simulink model "FlightSimulation"  (R2025b)
settings: Solver=ode3  StartTime=0.0  StopTime=100  FixedStep=params.time.dt  RelTol=1e-3
values from neighbouring files (symbols this model uses):
  launch_ECEF_m = lla2ecef(launchLLA)    [RunSim.m]    (also in RunSimulink.m)
  launchAlt = 180    [RunSim.m]    (also in RunSimulink.m = 10)
  launchLLA = [launchLat, launchLon, launchAlt]    [RunSim.m]    (also in RunSimulink.m)
  q = q / norm(q)    [CorrectQuaternionKinematics.m]    (also in solveLQR.m = 0.5*rho*vel^2)
  q_TB_0 = dcm2quat(R_TB_0)    [RunSimulink.m]
  w_ib_x = 0.00    (= 0)    [RunSim.m]    (also in RunSimulink.m = 1e-10)
  w_ib_y = 0.00    (= 0)    [RunSim.m]    (also in RunSimulink.m = 1e-10)
  w_ib_z = 0.00    (= 0)    [RunSim.m]    (also in RunSimulink.m = 1e-10)
undefined symbols (not defined in the file or in its folder): Earth, F, kfConsts, kfErrInds, kfInds, launchGeoidHeight, Light, MIL, nav_covs, nav_state, params, WGS84, WMM2025
libraries: simulink x6, aerolibatmos2 x5, aerolibgravity2 x3, aerolib6dof2 x1, aerolibwind2 x1, simulink_extras x1, matrix_library x1, aerolibtransform2 x1, lib_utils x1
(part 1 of 2)
settings Model: Creator=pearsdj1  LastModifiedBy=abhay

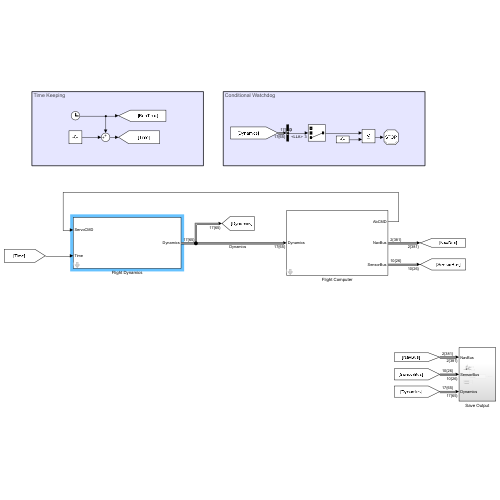
[thumbnail: Simulink's stored preview of the top-level diagram]
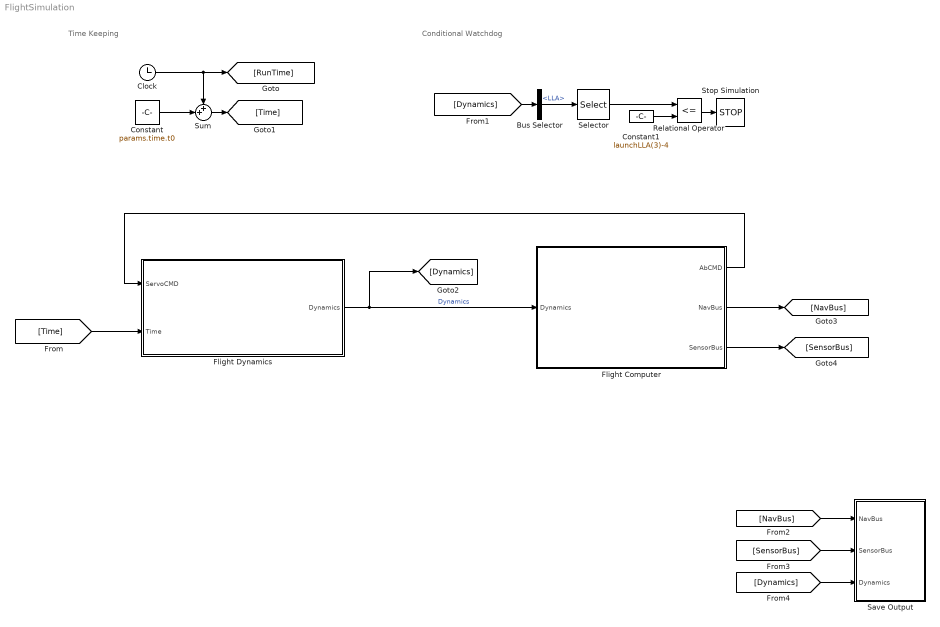
== system FlightSimulation ==
  note: Time Keeping
  note: Conditional Watchdog
  Bus Selector : BusSelector  OutputSignals=LLA
  Clock : Clock
  Constant : Constant  Value=params.time.t0
  Constant1 : Constant  Value=launchLLA(3)-4
  Flight Computer : Subsystem  mask{navParams=params.navParams, navInds=params.navInds, navConst=params.navConst, const=params.const, time=params.time}
      mask prompts: navParams "Navigator Params"; navInds "Navigator Indices"; navConst "Navigator Constants"; const "Constants"
      mask DialogControl DescGroupVar Prompt: Flight Computer
      mask DialogControl DescTextVar Prompt: Here lies the flight computer, with stuff and things ya'know
      mask DialogControl ParameterGroupVar Prompt: Navigator Parameters
  Flight Dynamics : Subsystem  mask{MotorModel=params.MotorModel, kins=params.kins, AeroModel=params.AeroModel, const=params.const}
      mask prompts: MotorModel "Motor Model"; kins "Kinematic Model"; AeroModel "Aerodynamic Model"; const "Constants"
      mask DialogControl DescGroupVar Prompt: Flight Dynamics
      mask DialogControl DescTextVar Prompt: Here be the dynamics of Sir Archimedes, according to all known laws of aviation...
  Relational Operator : RelationalOperator  Operator=<=  OutDataTypeStr=boolean  RndMeth=Simplest  InputSameDT=off
  Save Output : Subsystem
  Selector : Selector  InputPortWidth=3  IndexOptions=Index vector (dialog)  Indices=3  OutputSizes=1
  Stop Simulation : Stop
  Sum : Sum  Inputs=++|
  wires:
  Constant/1 -> Sum/2
  Clock/1 -> Sum/1, [RunTime]
  Sum/1 -> [Time]
  Flight Dynamics/1(Dynamics) -> [Dynamics], Flight Computer/1(Dynamics)  "Dynamics"
  Flight Computer/2(NavBus) -> [NavBus]
  Flight Computer/3(SensorBus) -> [SensorBus]
  [Time] -> Flight Dynamics/2(Time)
  Flight Computer/1(AbCMD) -> Flight Dynamics/1(ServoCMD)
  Constant1/1 -> Relational Operator/2
  [Dynamics] -> Bus Selector/1
  Bus Selector/1 -> Selector/1  "<LLA>"
  Selector/1 -> Relational Operator/1
  Relational Operator/1 -> Stop Simulation/1
  [NavBus] -> Save Output/1(NavBus)
  [SensorBus] -> Save Output/2(SensorBus)
  [Dynamics] -> Save Output/3(Dynamics)

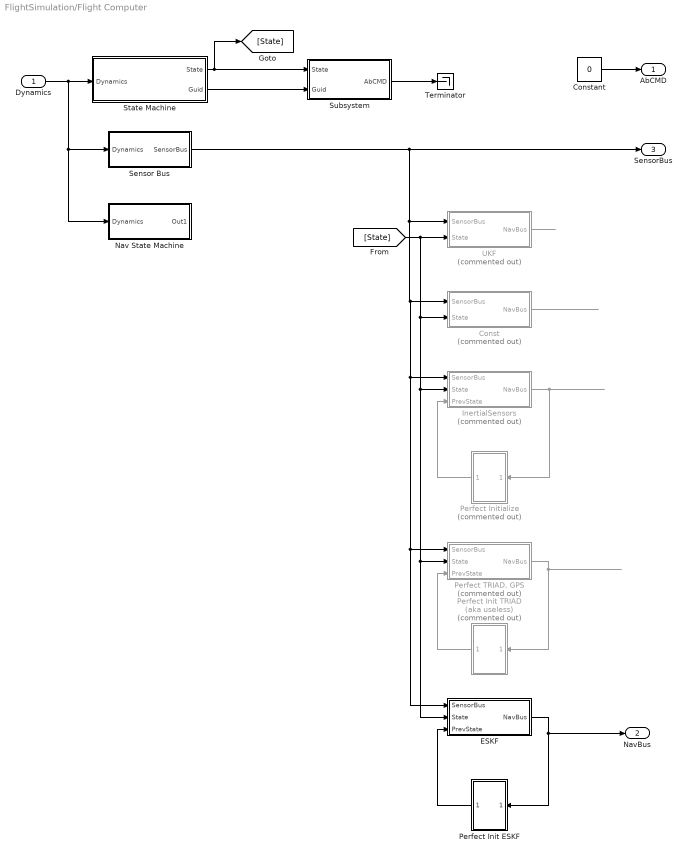
== system FlightSimulation/Flight Computer ==
  Dynamics : Inport
  Const : Subsystem  Commented=on
  Constant : Constant  Value=0
  ESKF : Subsystem
  InertialSensors : Subsystem  Commented=on
  Nav State Machine : Subsystem
  Perfect Init ESKF : Subsystem
  Perfect Init TRIAD (aka useless) : Subsystem  Commented=on
  Perfect Initialize : Subsystem  Commented=on
  "Perfect TRIAD, GPS" : Subsystem  Commented=on
  Sensor Bus : Subsystem
  State Machine : Subsystem
  Subsystem : Subsystem
  Terminator : Terminator
  UKF : Subsystem  Commented=on  TreatAsAtomicUnit=on  SystemSampleTime=time.navDt
  AbCMD : Outport
  NavBus : Outport  Port=2
  SensorBus : Outport  Port=3
  wires:
  Dynamics/1 -> Nav State Machine/1(Dynamics), Sensor Bus/1(Dynamics), State Machine/1(Dynamics)
  State Machine/1(State) -> [State], Subsystem/1(State)
  Constant/1 -> AbCMD/1
  Subsystem/1(AbCMD) -> Terminator/1
  State Machine/2(Guid) -> Subsystem/2(Guid)
  Sensor Bus/1(SensorBus) -> ESKF/1(SensorBus), "Perfect TRIAD, GPS"/1(SensorBus), InertialSensors/1(SensorBus), Const/1(SensorBus), UKF/1(SensorBus), SensorBus/1
  [State] -> ESKF/2(State), "Perfect TRIAD, GPS"/2(State), InertialSensors/2(State), Const/2(State), UKF/2(State)
  UKF/1(NavBus) -> ?
  Const/1(NavBus) -> ?
  InertialSensors/1(NavBus) -> Perfect Initialize/1(In1)
  Perfect Initialize/1(Out1) -> InertialSensors/3(PrevState)
  "Perfect TRIAD, GPS"/1(NavBus) -> Perfect Init TRIAD (aka useless)/1(NavBus)
  Perfect Init TRIAD (aka useless)/1(PrevState) -> "Perfect TRIAD, GPS"/3(PrevState)
  ESKF/1(NavBus) -> NavBus/1, Perfect Init ESKF/1(NavBus)
  Perfect Init ESKF/1(PrevState) -> ESKF/3(PrevState)

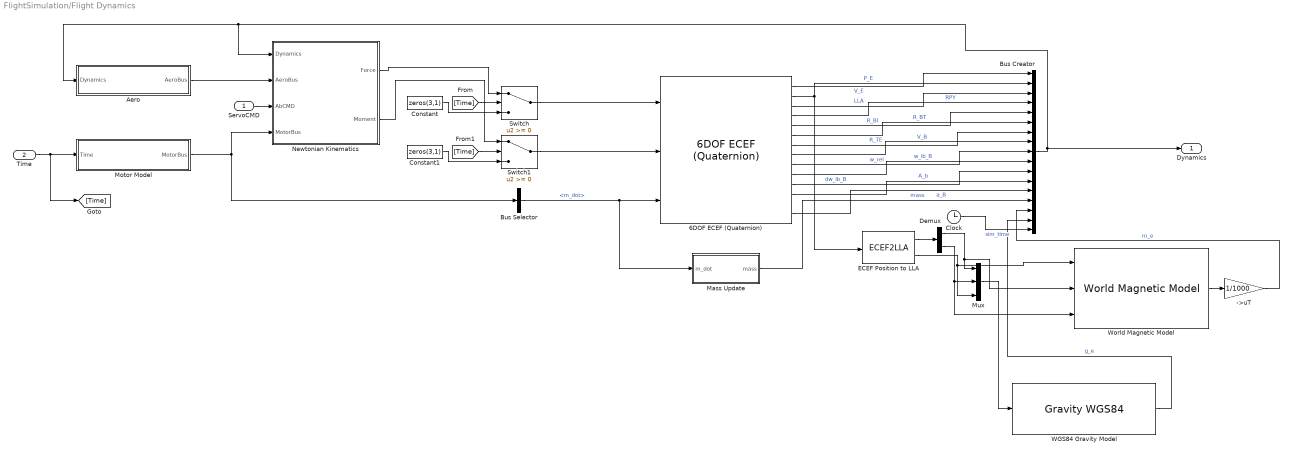
== system FlightSimulation/Flight Dynamics ==
  ServoCMD : Inport
  Time : Inport  Port=2
  ->uT : Gain  Gain=1/1000
  6DOF ECEF (Quaternion) : aerolib6dof2/6DOF ECEF (Quaternion)  units=Metric (MKS)  mtype=Simple Variable  xg_0=launchLLA  Vm_0=v_0_B  eul_0=eul_0  pm_0=[w_ib_x; w_ib_y; w_ib_z]  mass_0=kins.m_0 + MotorModel.emptyWt + MotorModel.propWt  mass_e=kins.m_0 + MotorModel.emptyWt  mass_f=kins.m_0 + MotorModel.emptyWt + MotorModel.propWt  inertia=eye(3)  inertia_e=kins.I_empty  inertia_f=kins.I_full  vre_flag=off  abi_flag=on  ptype=Earth (WGS84)  R=6378137  F=1/298.257223563  w_E=7292115e-11  angle_in=Internal  LPM0=0  quat_statename=''  pm_statename=''  Vm_statename=''  posfixedframe_statename=''  posinertial_statename=''  LPM_statename=''  mass_statename=''
  Aero : Subsystem
  Bus Creator : BusCreator  Inputs=17
  Bus Selector : BusSelector  OutputSignals=m_dot
  Clock : Clock
  Constant : Constant  Value=zeros(3,1)
  Constant1 : Constant  Value=zeros(3,1)
  Demux : Demux  Outputs=2
  ECEF Position to LLA : ECEF2LLA
  Mass Update : Subsystem
  Motor Model : Subsystem
  Mux : Mux  Inputs=3
  Newtonian Kinematics : Subsystem
  Switch : Switch  SaturateOnIntegerOverflow=off  InputSameDT=off
  Switch1 : Switch  SaturateOnIntegerOverflow=off  InputSameDT=off
  "WGS84 Gravity Model  " : GravityWGS84
  World Magnetic Model : aerolibgravity2/World Magnetic Model  model=WMM2025 (2025-2030)  customFile='WMM2025.COF'  units=Metric (MKS)  time_in=off  month=January  day=1  year=2026  action=Error  h_out=off  dec_out=off  inc_out=off  ti_out=off
  Dynamics : Outport
  wires:
  Aero/1(AeroBus) -> Newtonian Kinematics/2(AeroBus)
  Constant/1 -> Switch/3
  [Time] -> Switch/2
  Switch/1 -> 6DOF ECEF (Quaternion)/1
  Newtonian Kinematics/1(Force) -> Switch/1
  [Time] -> Switch1/2
  Newtonian Kinematics/2(Moment) -> Switch1/1
  Constant1/1 -> Switch1/3
  ServoCMD/1 -> Newtonian Kinematics/3(AbCMD)
  Time/1 -> Motor Model/1(Time), [Time]
  Motor Model/1(MotorBus) -> Bus Selector/1, Newtonian Kinematics/4(MotorBus)
  Switch1/1 -> 6DOF ECEF (Quaternion)/2
  Bus Selector/1 -> Mass Update/1(m_dot), 6DOF ECEF (Quaternion)/3  "<m_dot>"
  6DOF ECEF (Quaternion)/1 -> Bus Creator/1  "V_E"
  6DOF ECEF (Quaternion)/2 -> ECEF Position to LLA/1, Bus Creator/2  "P_E"
  6DOF ECEF (Quaternion)/3 -> Bus Creator/3  "LLA"
  6DOF ECEF (Quaternion)/4 -> Bus Creator/4  "RPY"
  6DOF ECEF (Quaternion)/5 -> Bus Creator/5  "R_BI"
  6DOF ECEF (Quaternion)/6 -> Bus Creator/6  "R_BT"
  6DOF ECEF (Quaternion)/7 -> Bus Creator/7  "R_TE"
  6DOF ECEF (Quaternion)/8 -> Bus Creator/8  "V_B"
  6DOF ECEF (Quaternion)/9 -> Bus Creator/9  "w_rel"
  6DOF ECEF (Quaternion)/10 -> Bus Creator/10  "w_ib_B"
  6DOF ECEF (Quaternion)/11 -> Bus Creator/11  "dw_ib_B"
  6DOF ECEF (Quaternion)/12 -> Bus Creator/12  "A_b"
  6DOF ECEF (Quaternion)/14 -> Bus Creator/13  "a_B"
  Mass Update/1(mass) -> Bus Creator/14  "mass"
  Bus Creator/1 -> Newtonian Kinematics/1(Dynamics), Aero/1(Dynamics), Dynamics/1
  ECEF Position to LLA/2 -> World Magnetic Model/1, Mux/3
  ECEF Position to LLA/1 -> Demux/1
  Demux/1 -> World Magnetic Model/2, Mux/1
  Demux/2 -> World Magnetic Model/3, Mux/2
  Mux/1 -> "WGS84 Gravity Model  "/1
  World Magnetic Model/1 -> ->uT/1
  ->uT/1 -> Bus Creator/15  "m_e"
  "WGS84 Gravity Model  "/1 -> Bus Creator/16  "g_e"
  Clock/1 -> Bus Creator/17  "sim_time"

== system FlightSimulation/Save Output ==
  NavBus : Inport
  SensorBus : Inport  Port=2
  Dynamics : Inport  Port=3
  Bus Selector : BusSelector  OutputSignals=P_E
  Digital Clock : DigitalClock
  ECEF To ECI : lib_utils/ECEF To ECI  Commented=on  SystemSampleTime=-1  VariantActivationTime=update diagram  EmptyChoice=off  PassThrough=off  PassThroughVariantControl=(default)  EmptyChoiceVariantControl=(default)  AllowFlexibleInterface=on  Latency=0  AutoFrameSizeCalculation=off
  To File : ToFile  Filename=dynamics.mat  SaveFormat=Timeseries
  To Workspace1 : ToWorkspace  VariableName=DynamicsBus  SaveFormat=Timeseries  SampleTime=-1
  To Workspace10 : ToWorkspace  VariableName=SensorBus  SaveFormat=Timeseries  SampleTime=-1
  To Workspace11 : ToWorkspace  Commented=on  VariableName=P_I  SaveFormat=Timeseries  SampleTime=-1
  To Workspace9 : ToWorkspace  VariableName=NavBus  SaveFormat=Timeseries  SampleTime=-1
  wires:
  Bus Selector/1 -> ECEF To ECI/2  "<P_E>"
  NavBus/1 -> To Workspace9/1
  SensorBus/1 -> To Workspace10/1
  Digital Clock/1 -> ECEF To ECI/1
  ECEF To ECI/1 -> To Workspace11/1
  Dynamics/1 -> To Workspace1/1, To File/1, Bus Selector/1

== system FlightSimulation/Flight Computer/Const ==
  note: Note: These functions do nothing, but are to trick matlab into calcualting every timestep
  SensorBus : Inport
  State : Inport  Port=2
  Bus Creator : BusCreator  Inputs=2
  Bus Selector : BusSelector  OutputSignals=ICM20948.w_ib_B_true
  Constant : Constant  Value=q_TB_0'
  MATLAB Function : MATLAB Function  TreatAsAtomicUnit=on
  MATLAB Function1 : MATLAB Function  TreatAsAtomicUnit=on
  Terminator : Terminator
  Vector Concatenate : Concatenate
  NavBus : Outport
  wires:
  SensorBus/1 -> Bus Selector/1
  Constant/1 -> Vector Concatenate/1
  Vector Concatenate/1 -> Bus Creator/1  "x"
  MATLAB Function/1(y) -> Vector Concatenate/2
  Bus Selector/1 -> MATLAB Function1/1(u), MATLAB Function/1(u)  "<w_ib_B_true>"
  MATLAB Function1/1(y) -> Bus Creator/2  "P"
  Bus Creator/1 -> NavBus/1

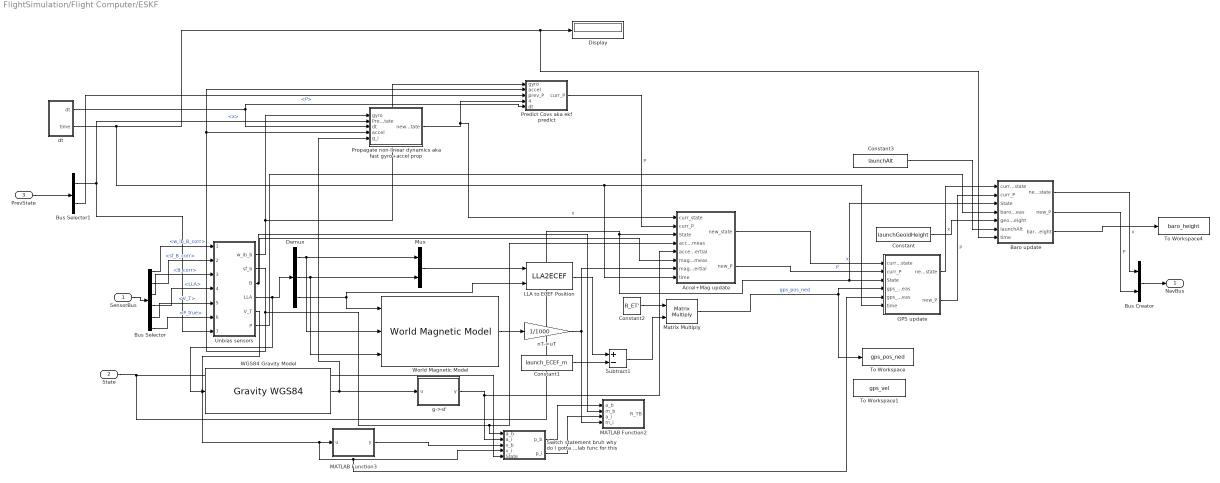
== system FlightSimulation/Flight Computer/ESKF ==
  SensorBus : Inport
  State : Inport  Port=2
  PrevState : Inport  Port=3
  Accel+Mag update : MATLAB Function  TreatAsAtomicUnit=on
  Baro update : MATLAB Function  TreatAsAtomicUnit=on
  Bus Creator : BusCreator  Inputs=2
  Bus Selector : BusSelector  OutputSignals=ICM20948.w_ib_B_corr,ICM20948.sf_B_corr,MMC5983.B_corr,MAX10S.LLA,MAX10S.V_T,LPS22.P_true
  Bus Selector1 : BusSelector  OutputSignals=x,P
  Constant : Constant  Value=launchGeoidHeight
  Constant1 : Constant  Value=launch_ECEF_m
  Constant2 : Constant  Value=R_ET'
  Constant3 : Constant  Value=launchAlt
  Demux : Demux  Outputs=3
  Display : Display
  GPS update : MATLAB Function  TreatAsAtomicUnit=on
  LLA to ECEF Position : LLA2ECEF
  MATLAB Function2 : MATLAB Function  TreatAsAtomicUnit=on
  MATLAB Function3 : MATLAB Function  TreatAsAtomicUnit=on
  Matrix Multiply : Product  Multiplication=Matrix(*)
  Mux : Mux  Inputs=2
  Predict Covs aka ekf predict : MATLAB Function  TreatAsAtomicUnit=on
  Propagate non-linear dynamics aka fast gyro+accel prop : MATLAB Function  TreatAsAtomicUnit=on
  Subtract1 : Sum  Inputs=+-
  Switch statement bruh why do i gotta make a matlab func for this : MATLAB Function  TreatAsAtomicUnit=on
  To Workspace : ToWorkspace  VariableName=gps_pos_ned  SaveFormat=Timeseries  SampleTime=-1
  To Workspace1 : ToWorkspace  VariableName=gps_vel  SaveFormat=Timeseries  SampleTime=-1
  To Workspace4 : ToWorkspace  VariableName=baro_height  SaveFormat=Timeseries  SampleTime=-1
  Unbias sensors : MATLAB Function  TreatAsAtomicUnit=on
  "WGS84 Gravity Model  " : GravityWGS84
  World Magnetic Model : aerolibgravity2/World Magnetic Model  model=WMM2025 (2025-2030)  customFile='WMM2025.COF'  units=Metric (MKS)  time_in=off  month=January  day=1  year=2025  action=Error  h_out=off  dec_out=off  inc_out=off  ti_out=off
  dt : Subsystem
  g->sf : MATLAB Function  TreatAsAtomicUnit=on
  nT->uT : Gain  Gain=1/1000
  NavBus : Outport
  wires:
  SensorBus/1 -> Bus Selector/1
  Demux/3 -> LLA to ECEF Position/2, World Magnetic Model/1
  Bus Selector1/2 -> Predict Covs aka ekf predict/3(prev_P)  "<P>"
  Demux/1 -> Mux/1, World Magnetic Model/2
  Demux/2 -> Mux/2, World Magnetic Model/3
  "WGS84 Gravity Model  "/1 -> Propagate non-linear dynamics aka fast gyro+accel prop/5(g_i), g->sf/1(u)
  Mux/1 -> LLA to ECEF Position/1
  World Magnetic Model/1 -> nT->uT/1
  g->sf/1(y) -> Switch statement bruh why do i gotta make a matlab func for this/2(a_i), Accel+Mag update/5(accel_inertial)
  LLA to ECEF Position/1 -> Subtract1/1
  Constant1/1 -> Subtract1/2
  Constant2/1 -> Matrix Multiply/1
  PrevState/1 -> Bus Selector1/1
  Matrix Multiply/1 -> To Workspace/1, GPS update/4(gps_pos_meas)  "gps_pos_ned"
  Bus Creator/1 -> NavBus/1
  Switch statement bruh why do i gotta make a matlab func for this/1(p_b) -> MATLAB Function2/1(a_b)
  Switch statement bruh why do i gotta make a matlab func for this/2(p_i) -> MATLAB Function2/3(a_i)
  MATLAB Function3/1(y) -> Switch statement bruh why do i gotta make a matlab func for this/3(v_b)
  State/1 -> Switch statement bruh why do i gotta make a matlab func for this/5(State), Baro update/3(State), GPS update/3(State), Accel+Mag update/3(State)
  Bus Selector/1 -> Unbias sensors/1(w_ib_b_biased)  "<w_ib_B_corr>"
  Propagate non-linear dynamics aka fast gyro+accel prop/1(newState) -> Predict Covs aka ekf predict/4(curr_state), Accel+Mag update/1(curr_state)  "x"
  Bus Selector1/1 -> Unbias sensors/7(prev_state), Propagate non-linear dynamics aka fast gyro+accel prop/2(PrevState)  "<x>"
  dt/1(dt) -> Propagate non-linear dynamics aka fast gyro+accel prop/3(dt), Predict Covs aka ekf predict/5(dt)
  Predict Covs aka ekf predict/1(curr_P) -> Accel+Mag update/2(curr_P)  "P"
  nT->uT/1 -> Accel+Mag update/7(mag_inertial), MATLAB Function2/4(m_i)
  Accel+Mag update/1(new_state) -> GPS update/1(curr_state)  "x"
  Accel+Mag update/2(new_P) -> GPS update/2(curr_P)  "P"
  Subtract1/1 -> Matrix Multiply/2
  dt/2(time) -> GPS update/6(time), Accel+Mag update/8(time), Baro update/7(time), Display/1
  Bus Selector/6 -> Unbias sensors/6(P_biased)  "<P_true>"
  Constant/1 -> Baro update/5(geoid_height)
  Baro update/3(baro_height) -> To Workspace4/1
  Constant3/1 -> Baro update/6(launchAlt)
  Unbias sensors/1(w_ib_b) -> Predict Covs aka ekf predict/1(gyro), Propagate non-linear dynamics aka fast gyro+accel prop/1(gyro)
  Bus Selector/2 -> Unbias sensors/2(sf_b_biased)  "<sf_B_corr>"
  Unbias sensors/2(sf_b) -> Predict Covs aka ekf predict/2(accel), Propagate non-linear dynamics aka fast gyro+accel prop/4(accel), Accel+Mag update/4(accel_meas), Switch statement bruh why do i gotta make a matlab func for this/1(a_b)
  Unbias sensors/3(B) -> MATLAB Function2/2(m_b), Accel+Mag update/6(mag_meas)
  Bus Selector/4 -> Unbias sensors/4(LLA_biased)  "<LLA>"
  Unbias sensors/4(LLA) -> "WGS84 Gravity Model  "/1, Demux/1
  Bus Selector/5 -> Unbias sensors/5(V_T_biased)  "<V_T>"
  Unbias sensors/5(V_T) -> GPS update/5(gps_vel_meas), Switch statement bruh why do i gotta make a matlab func for this/4(v_i), MATLAB Function3/1(u)
  Unbias sensors/6(P) -> Baro update/4(baro_meas)
  GPS update/1(new_state) -> Baro update/1(curr_state)  "x"
  GPS update/2(new_P) -> Baro update/2(curr_P)  "P"
  Bus Selector/3 -> Unbias sensors/3(B_biased)  "<B_corr>"
  Baro update/2(new_P) -> Bus Creator/2  "P"
  Baro update/1(new_state) -> Bus Creator/1  "x"

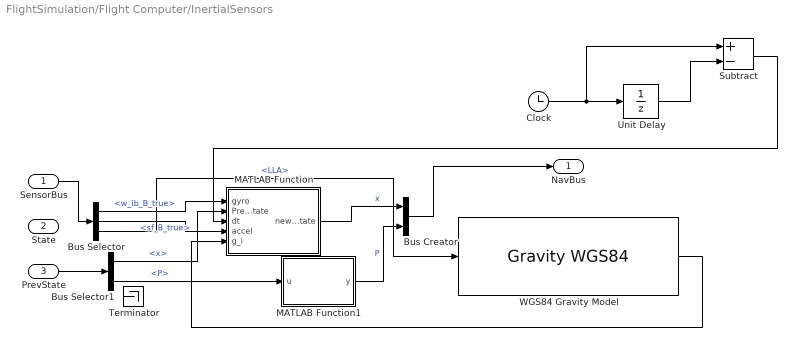
== system FlightSimulation/Flight Computer/InertialSensors ==
  SensorBus : Inport
  State : Inport  Port=2
  PrevState : Inport  Port=3
  Bus Creator : BusCreator  Inputs=2
  Bus Selector : BusSelector  OutputSignals=ICM20948.w_ib_B_true,ICM20948.sf_B_true,MAX10S.LLA
  Bus Selector1 : BusSelector  OutputSignals=x,P
  Clock : Clock
  MATLAB Function : MATLAB Function  TreatAsAtomicUnit=on
  MATLAB Function1 : MATLAB Function  TreatAsAtomicUnit=on
  Subtract : Sum  Inputs=+-
  Terminator : Terminator
  Unit Delay : UnitDelay  SampleTime=-1  HasFrameUpgradeWarning=on
  "WGS84 Gravity Model  " : GravityWGS84
  NavBus : Outport
  wires:
  SensorBus/1 -> Bus Selector/1
  MATLAB Function/1(newState) -> Bus Creator/1  "x"
  Bus Selector/1 -> MATLAB Function/1(gyro)  "<w_ib_B_true>"
  MATLAB Function1/1(y) -> Bus Creator/2  "P"
  Bus Creator/1 -> NavBus/1
  Clock/1 -> Unit Delay/1, Subtract/1
  Unit Delay/1 -> Subtract/2
  Subtract/1 -> MATLAB Function/3(dt)
  PrevState/1 -> Bus Selector1/1
  Bus Selector1/1 -> MATLAB Function/2(PrevState)  "<x>"
  Bus Selector1/2 -> MATLAB Function1/1(u)  "<P>"
  Bus Selector/3 -> "WGS84 Gravity Model  "/1  "<LLA>"
  Bus Selector/2 -> MATLAB Function/4(accel)  "<sf_B_true>"
  "WGS84 Gravity Model  "/1 -> MATLAB Function/5(g_i)

== system FlightSimulation/Flight Computer/Nav State Machine ==
  Dynamics : Inport
  Bus Selector : BusSelector  OutputSignals=A_b,LLA,V_B
  Chart : Stateflow chart  TreatAsAtomicUnit=on
  Out1 : Outport
  wires:
  Dynamics/1 -> Bus Selector/1

== system FlightSimulation/Flight Computer/Perfect Init ESKF ==
  NavBus : Inport
  Bus Creator : BusCreator  Inputs=2
  Bus Selector : BusSelector  OutputSignals=x,P
  Constant1 : Constant  Value=nav_state
  Constant2 : Constant  Value=nav_covs
  Delay : Delay  DelayLength=1  InitialConditionSource=Input port
      settings: InputPortMap=u0,p4
  Delay1 : Delay  DelayLength=1  InitialConditionSource=Input port
      settings: InputPortMap=u0,p4
  PrevState : Outport
  wires:
  Bus Selector/1 -> Delay/1  "<x>"
  Delay1/1 -> Bus Creator/2  "P"
  Constant1/1 -> Delay/2
  NavBus/1 -> Bus Selector/1
  Delay/1 -> Bus Creator/1  "x"
  Bus Creator/1 -> PrevState/1
  Bus Selector/2 -> Delay1/1  "<P>"
  Constant2/1 -> Delay1/2

== system FlightSimulation/Flight Computer/Perfect Init TRIAD (aka useless) ==
  NavBus : Inport
  Bus Creator : BusCreator  Inputs=2
  Bus Selector : BusSelector  OutputSignals=x,P
  Constant1 : Constant  Value=[q_TB_0'; zeros(19, 1)]
  Constant2 : Constant  Value=eye(22)
  Delay : Delay  DelayLength=1  InitialConditionSource=Input port
      settings: InputPortMap=u0,p4
  Delay1 : Delay  DelayLength=1  InitialConditionSource=Input port
      settings: InputPortMap=u0,p4
  PrevState : Outport
  wires:
  Bus Selector/1 -> Delay/1  "<x>"
  Delay1/1 -> Bus Creator/2  "P"
  Constant1/1 -> Delay/2
  NavBus/1 -> Bus Selector/1
  Delay/1 -> Bus Creator/1  "x"
  Bus Creator/1 -> PrevState/1
  Bus Selector/2 -> Delay1/1  "<P>"
  Constant2/1 -> Delay1/2

== system FlightSimulation/Flight Computer/Perfect Initialize ==
  In1 : Inport
  Bus Creator : BusCreator  Inputs=2
  Bus Selector : BusSelector  OutputSignals=x,P
  Constant1 : Constant  Value=[q_TB_0'; zeros(19, 1)]
  Constant2 : Constant  Value=eye(22)
  Delay : Delay  DelayLength=1  InitialConditionSource=Input port
      settings: InputPortMap=u0,p4
  Delay1 : Delay  DelayLength=1  InitialConditionSource=Input port
      settings: InputPortMap=u0,p4
  Out1 : Outport
  wires:
  Bus Selector/1 -> Delay/1  "<x>"
  Delay1/1 -> Bus Creator/2  "P"
  Constant1/1 -> Delay/2
  In1/1 -> Bus Selector/1
  Delay/1 -> Bus Creator/1  "x"
  Bus Creator/1 -> Out1/1
  Bus Selector/2 -> Delay1/1  "<P>"
  Constant2/1 -> Delay1/2

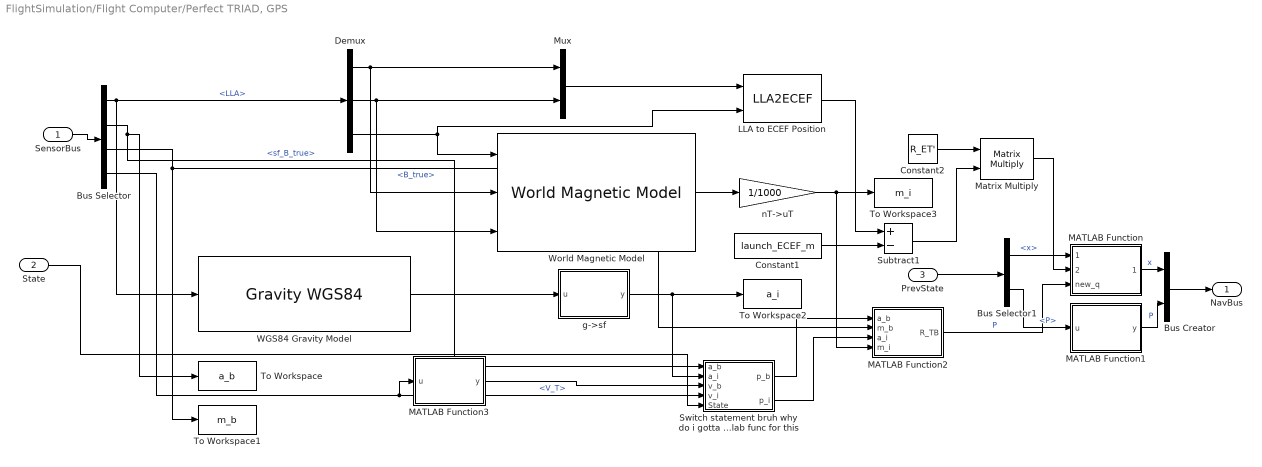
== system FlightSimulation/Flight Computer/Perfect TRIAD, GPS ==
  SensorBus : Inport
  State : Inport  Port=2
  PrevState : Inport  Port=3
  Bus Creator : BusCreator  Inputs=2
  Bus Selector : BusSelector  OutputSignals=MAX10S.LLA,ICM20948.sf_B_true,MMC5983.B_true,MAX10S.V_T
  Bus Selector1 : BusSelector  OutputSignals=x,P
  Constant1 : Constant  Value=launch_ECEF_m
  Constant2 : Constant  Value=R_ET'
  Demux : Demux  Outputs=3
  LLA to ECEF Position : LLA2ECEF
  MATLAB Function : MATLAB Function  TreatAsAtomicUnit=on
  MATLAB Function1 : MATLAB Function  TreatAsAtomicUnit=on
  MATLAB Function2 : MATLAB Function  TreatAsAtomicUnit=on
  MATLAB Function3 : MATLAB Function  TreatAsAtomicUnit=on
  Matrix Multiply : Product  Multiplication=Matrix(*)
  Mux : Mux  Inputs=2
  Subtract1 : Sum  Inputs=+-
  Switch statement bruh why do i gotta make a matlab func for this : MATLAB Function  TreatAsAtomicUnit=on
  To Workspace : ToWorkspace  VariableName=a_b  SaveFormat=Timeseries  SampleTime=-1
  To Workspace1 : ToWorkspace  VariableName=m_b  SaveFormat=Timeseries  SampleTime=-1
  To Workspace2 : ToWorkspace  VariableName=a_i  SaveFormat=Timeseries  SampleTime=-1
  To Workspace3 : ToWorkspace  VariableName=m_i  SaveFormat=Timeseries  SampleTime=-1
  "WGS84 Gravity Model  " : GravityWGS84
  World Magnetic Model : aerolibgravity2/World Magnetic Model  model=WMM2025 (2025-2030)  customFile='WMM2025.COF'  units=Metric (MKS)  time_in=off  month=January  day=1  year=2025  action=Error  h_out=off  dec_out=off  inc_out=off  ti_out=off
  g->sf : MATLAB Function  TreatAsAtomicUnit=on
  nT->uT : Gain  Gain=1/1000
  NavBus : Outport
  wires:
  SensorBus/1 -> Bus Selector/1
  Bus Selector/1 -> Demux/1, "WGS84 Gravity Model  "/1  "<LLA>"
  Bus Selector/3 -> MATLAB Function2/2(m_b), To Workspace1/1  "<B_true>"
  Bus Selector/2 -> Switch statement bruh why do i gotta make a matlab func for this/1(a_b), To Workspace/1  "<sf_B_true>"
  Demux/3 -> LLA to ECEF Position/2, World Magnetic Model/1
  Bus Selector1/2 -> MATLAB Function1/1(u)  "<P>"
  Demux/1 -> Mux/1, World Magnetic Model/2
  Demux/2 -> Mux/2, World Magnetic Model/3
  "WGS84 Gravity Model  "/1 -> g->sf/1(u)
  Mux/1 -> LLA to ECEF Position/1
  World Magnetic Model/1 -> nT->uT/1
  g->sf/1(y) -> Switch statement bruh why do i gotta make a matlab func for this/2(a_i), To Workspace2/1
  LLA to ECEF Position/1 -> Subtract1/1
  nT->uT/1 -> MATLAB Function2/4(m_i), To Workspace3/1
  MATLAB Function2/1(R_TB) -> MATLAB Function/3(new_q)  "P"
  Constant1/1 -> Subtract1/2
  Constant2/1 -> Matrix Multiply/1
  Subtract1/1 -> Matrix Multiply/2
  PrevState/1 -> Bus Selector1/1
  Matrix Multiply/1 -> MATLAB Function/2(new_pos)
  Bus Selector1/1 -> MATLAB Function/1(PrevState)  "<x>"
  MATLAB Function/1(newState) -> Bus Creator/1  "x"
  MATLAB Function1/1(y) -> Bus Creator/2  "P"
  Bus Creator/1 -> NavBus/1
  Switch statement bruh why do i gotta make a matlab func for this/1(p_b) -> MATLAB Function2/1(a_b)
  Switch statement bruh why do i gotta make a matlab func for this/2(p_i) -> MATLAB Function2/3(a_i)
  MATLAB Function3/1(y) -> Switch statement bruh why do i gotta make a matlab func for this/3(v_b)
  Bus Selector/4 -> MATLAB Function3/1(u), Switch statement bruh why do i gotta make a matlab func for this/4(v_i)  "<V_T>"
  State/1 -> Switch statement bruh why do i gotta make a matlab func for this/5(State)

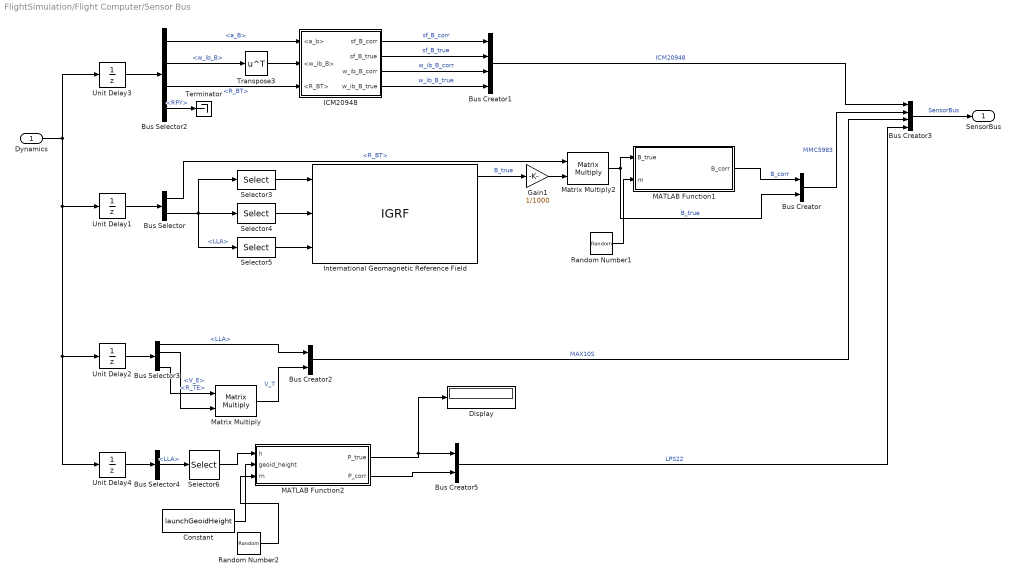
== system FlightSimulation/Flight Computer/Sensor Bus ==
  Dynamics : Inport
  Bus Creator : BusCreator  Inputs=2
  Bus Creator1 : BusCreator  Inputs=4
  Bus Creator2 : BusCreator  Inputs=2
  Bus Creator3 : BusCreator  Inputs=4
  Bus Creator5 : BusCreator  Inputs=2
  Bus Selector : BusSelector  OutputSignals=R_BT,LLA
  Bus Selector2 : BusSelector  OutputSignals=a_B,w_ib_B,R_BT,RPY
  Bus Selector3 : BusSelector  OutputSignals=LLA,V_E,R_BT,R_TE
  Bus Selector4 : BusSelector  OutputSignals=LLA
  Constant : Constant  Value=launchGeoidHeight
  Display : Display
  Gain1 : Gain  Gain=1/1000
  ICM20948 : Subsystem
  International Geomagnetic Reference Field : IGRF  time_in=off  month=January  day=1  sv_out=off
      settings: AttributesFormatString=%<generation>
  MATLAB Function1 : MATLAB Function  TreatAsAtomicUnit=on
  MATLAB Function2 : MATLAB Function  TreatAsAtomicUnit=on
  Matrix Multiply : Product  Multiplication=Matrix(*)
  Matrix Multiply2 : Product  Multiplication=Matrix(*)
  Random Number1 : RandomNumber
  Random Number2 : RandomNumber
  Selector3 : Selector  InputPortWidth=3  IndexOptions=Index vector (dialog)  Indices=3  OutputSizes=1
  Selector4 : Selector  InputPortWidth=3  IndexOptions=Index vector (dialog)  Indices=1  OutputSizes=1
  Selector5 : Selector  InputPortWidth=3  IndexOptions=Index vector (dialog)  Indices=2  OutputSizes=1
  Selector6 : Selector  InputPortWidth=3  IndexOptions=Index vector (dialog)  Indices=3  OutputSizes=1
  Terminator : Terminator
  Transpose3 : Math  Operator=transpose
  Unit Delay{1..4} (4 alike) : UnitDelay  SampleTime=-1  HasFrameUpgradeWarning=on
  SensorBus : Outport
  wires:
  Dynamics/1 -> Unit Delay4/1, Unit Delay2/1, Unit Delay1/1, Unit Delay3/1
  Bus Creator3/1 -> SensorBus/1  "SensorBus"
  Unit Delay3/1 -> Bus Selector2/1
  Bus Selector2/1 -> ICM20948/1(<a_b>)  "<a_B>"
  Bus Selector2/2 -> Transpose3/1  "<w_ib_B>"
  Bus Selector2/4 -> Terminator/1  "<RPY>"
  Bus Selector2/3 -> ICM20948/3(<R_BT>)  "<R_BT>"
  ICM20948/1(sf_B_corr) -> Bus Creator1/1  "sf_B_corr"
  ICM20948/2(sf_B_true) -> Bus Creator1/2  "sf_B_true"
  ICM20948/3(w_ib_B_corr) -> Bus Creator1/3  "w_ib_B_corr"
  ICM20948/4(w_ib_B_true) -> Bus Creator1/4  "w_ib_B_true"
  Bus Creator1/1 -> Bus Creator3/1  "ICM20948"
  Transpose3/1 -> ICM20948/2(<w_ib_B>)
  Unit Delay1/1 -> Bus Selector/1
  Selector3/1 -> International Geomagnetic Reference Field/1
  Bus Selector/2 -> Selector5/1, Selector3/1, Selector4/1  "<LLA>"
  Selector4/1 -> International Geomagnetic Reference Field/2
  Selector5/1 -> International Geomagnetic Reference Field/3
  MATLAB Function1/1(B_corr) -> Bus Creator/1  "B_corr"
  Bus Creator/1 -> Bus Creator3/2  "MMC5983"
  Bus Selector/1 -> Matrix Multiply2/1  "<R_BT>"
  Matrix Multiply2/1 -> Bus Creator/2, MATLAB Function1/1(B_true)  "B_true"
  International Geomagnetic Reference Field/1 -> Gain1/1  "B_true"
  Gain1/1 -> Matrix Multiply2/2
  Unit Delay2/1 -> Bus Selector3/1
  Bus Selector3/1 -> Bus Creator2/1  "<LLA>"
  Bus Creator2/1 -> Bus Creator3/3  "MAX10S"
  Unit Delay4/1 -> Bus Selector4/1
  Bus Selector4/1 -> Selector6/1  "<LLA>"
  Selector6/1 -> MATLAB Function2/1(h)
  MATLAB Function2/1(P_true) -> Display/1, Bus Creator5/1
  MATLAB Function2/2(P_corr) -> Bus Creator5/2
  Bus Creator5/1 -> Bus Creator3/4  "LPS22"
  Bus Selector3/2 -> Matrix Multiply/2  "<V_E>"
  Bus Selector3/4 -> Matrix Multiply/1  "<R_TE>"
  Matrix Multiply/1 -> Bus Creator2/2  "V_T"
  Constant/1 -> MATLAB Function2/2(geoid_height)
  Random Number1/1 -> MATLAB Function1/2(rn)
  Random Number2/1 -> MATLAB Function2/3(rn)

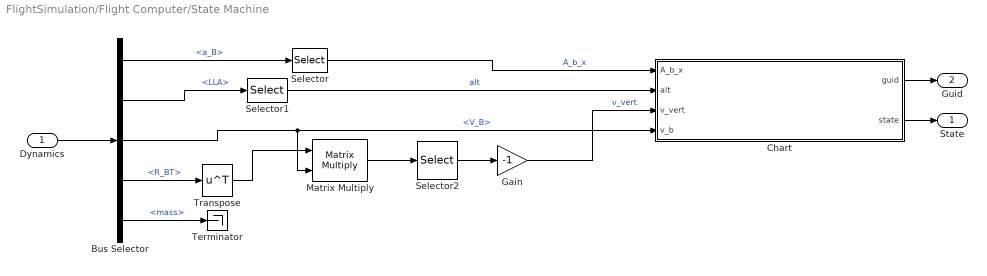
== system FlightSimulation/Flight Computer/State Machine ==
  Dynamics : Inport
  Bus Selector : BusSelector  OutputSignals=a_B,LLA,V_B,R_BT,mass
  Chart : Stateflow chart  TreatAsAtomicUnit=on
  Gain : Gain  Gain=-1
  Matrix Multiply : Product  Multiplication=Matrix(*)
  Selector : Selector  InputPortWidth=3  IndexOptions=Index vector (dialog)  Indices=1  OutputSizes=1
  Selector1 : Selector  InputPortWidth=3  IndexOptions=Index vector (dialog)  Indices=3  OutputSizes=1
  Selector2 : Selector  InputPortWidth=3  IndexOptions=Index vector (dialog)  Indices=3  OutputSizes=1
  Terminator : Terminator
  Transpose : Math  Operator=transpose
  State : Outport
  Guid : Outport  Port=2
  wires:
  Matrix Multiply/1 -> Selector2/1
  Bus Selector/2 -> Selector1/1  "<LLA>"
  Bus Selector/3 -> Matrix Multiply/2, Chart/4(v_b)  "<V_B>"
  Selector2/1 -> Gain/1
  Bus Selector/4 -> Transpose/1  "<R_BT>"
  Bus Selector/1 -> Selector/1  "<a_B>"
  Bus Selector/5 -> Terminator/1  "<mass>"
  Chart/2(state) -> State/1
  Dynamics/1 -> Bus Selector/1
  Chart/1(guid) -> Guid/1
  Selector/1 -> Chart/1(A_b_x)  "A_b_x"
  Selector1/1 -> Chart/2(alt)  "alt"
  Gain/1 -> Chart/3(v_vert)  "v_vert"
  Transpose/1 -> Matrix Multiply/1

== system FlightSimulation/Flight Computer/Subsystem ==
  State : Inport
  Guid : Inport  Port=2
  Compare To Constant : simulink/Logic and Bit Operations/Compare To Constant  relop===  const=1  OutDataTypeStr=boolean
  Constant : Constant  Value=0.75
  Constant1 : Constant  Value=0
  Switch1 : Switch  Criteria=u2 > Threshold  SaturateOnIntegerOverflow=off  InputSameDT=off
  Unit Delay : UnitDelay  SampleTime=-1  HasFrameUpgradeWarning=on
  AbCMD : Outport
  wires:
  Compare To Constant/1 -> Switch1/2
  Constant/1 -> Switch1/1
  Constant1/1 -> Switch1/3
  Switch1/1 -> AbCMD/1
  Unit Delay/1 -> Compare To Constant/1
  Guid/1 -> Unit Delay/1

== system FlightSimulation/Flight Computer/UKF ==
  SensorBus : Inport
  State : Inport  Port=2
  Compare To Constant : simulink/Logic and Bit Operations/Compare To Constant  relop===  const=1  OutDataTypeStr=boolean
  Delay One Step : Delay  DelayLength=1
  Delay1 : Delay  DelayLength=1  InitialConditionSource=Input port  InitialCondition=navParams.  ShowEnablePort=on
      settings: InputPortMap=u0,e6,p4
  Initialize Nav : Subsystem
  Prediction Step : Subsystem
  Update Step : Subsystem
  NavBus : Outport  OutDataTypeStr=Bus: navBus
  wires:
  SensorBus/1 -> Update Step/3(SensorBus), Prediction Step/2(SensorBus), Initialize Nav/1(SensorBus)
  Initialize Nav/1(initFlag) -> Compare To Constant/1
  Compare To Constant/1 -> Delay One Step/1
  Initialize Nav/2(NavBus) -> Delay1/3
  [navInit] -> Prediction Step/Enable
  Delay1/1 -> Prediction Step/1(NavBus)  "NavBus"
  Delay One Step/1 -> [navInit], Delay1/2
  [navInit] -> Update Step/Enable
  Update Step/1(navOut) -> NavBus/1, Delay1/1
  Prediction Step/1(navOut) -> Update Step/1(navBus)
  State/1 -> Update Step/2(State)

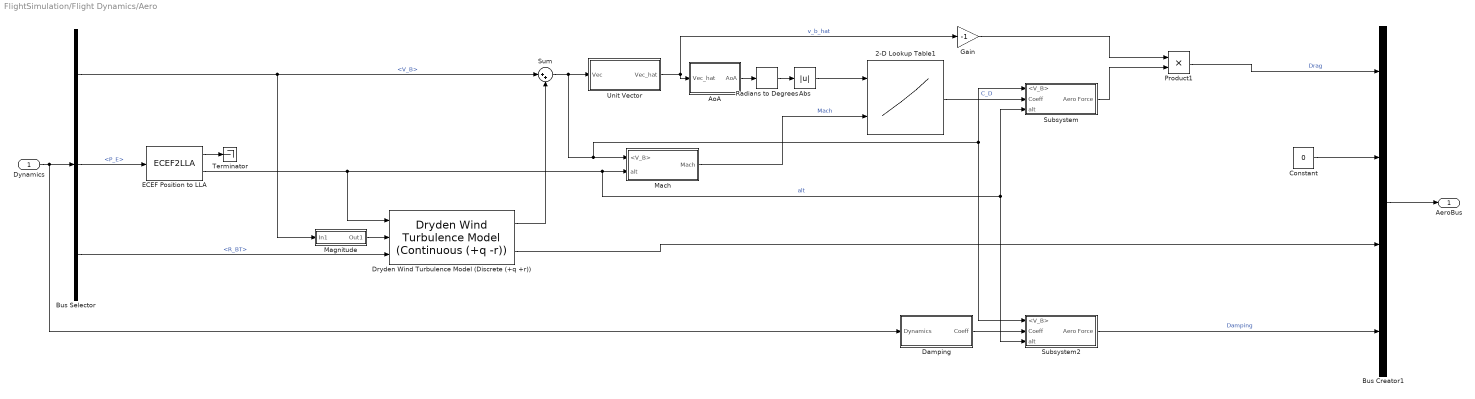
== system FlightSimulation/Flight Dynamics/Aero ==
  Dynamics : Inport
  2-D Lookup Table1 : Lookup_n-D  BreakpointsForDimension1=AeroModel.AoAs  BreakpointsForDimension2=AeroModel.MachNumbers  Table=AeroModel.CdGrid  ExtrapMethod=Clip  UseLastTableValue=on  ApplyAccurateEfficientRounding=on  InternalRulePriority=Speed  RndMeth=Simplest
      settings: InputPortMap=u0,u1
  Abs : Abs  SaturateOnIntegerOverflow=off
  AoA : Subsystem
  Bus Creator1 : BusCreator  Inputs=4
  Bus Selector : BusSelector  OutputSignals=V_B,P_E,R_BT
  Constant : Constant  Value=0
  Damping : Subsystem
  Dryden Wind Turbulence Model (Discrete (+q +r)) : aerolibwind2/Dryden Wind Turbulence Model  (Continuous (+q -r))  units=Metric (MKS)  spec=MIL-F-8785C  model=Discrete Dryden (+q +r)  W20=6  Wdeg=0  TurbProb=10^-2 - Light  L_high=533.4  Wingspan=0.127  ts=0.1  Seed=[23341 23342 23343 23344]  T_on=on
      settings: LibrarySourceBlock=|
      | aerolibwind2/Dryden Wind Turbulence Model
      | (Discrete (+q +r))
  ECEF Position to LLA : ECEF2LLA
  Gain : Gain  Gain=-1
  Mach : Subsystem
  Magnitude : Subsystem
  Product1 : Product
  Radians to Degrees : simulink_extras/Transformations/Radians to Degrees
  Subsystem : Subsystem
  Subsystem2 : Subsystem
  Sum : Sum  Inputs=|++
  Terminator : Terminator
  Unit Vector : Subsystem
  AeroBus : Outport
  wires:
  Dynamics/1 -> Damping/1(Dynamics), Bus Selector/1
  Bus Selector/2 -> ECEF Position to LLA/1  "<P_E>"
  ECEF Position to LLA/1 -> Terminator/1
  ECEF Position to LLA/2 -> Mach/2(alt), Subsystem/3(alt), Subsystem2/3(alt), Dryden Wind Turbulence Model (Discrete (+q +r))/1  "alt"
  Mach/1(Mach) -> 2-D Lookup Table1/2  "Mach"
  Unit Vector/1(Vec_hat) -> AoA/1(Vec_hat), Gain/1  "v_b_hat"
  AoA/1(AoA) -> Radians to Degrees/1
  Gain/1 -> Product1/1
  Product1/1 -> Bus Creator1/1  "Drag"
  Bus Creator1/1 -> AeroBus/1
  2-D Lookup Table1/1 -> Subsystem/2(Coeff)  "C_D"
  Subsystem/1(Aero Force) -> Product1/2
  Bus Selector/1 -> Magnitude/1(In1), Sum/1  "<V_B>"
  Magnitude/1(Out1) -> Dryden Wind Turbulence Model (Discrete (+q +r))/2
  Bus Selector/3 -> Dryden Wind Turbulence Model (Discrete (+q +r))/3  "<R_BT>"
  Sum/1 -> Subsystem/1(<V_B>), Subsystem2/1(<V_B>), Mach/1(<V_B>), Unit Vector/1(Vec)
  Dryden Wind Turbulence Model (Discrete (+q +r))/2 -> Bus Creator1/3
  Damping/1(Coeff) -> Subsystem2/2(Coeff)
  Subsystem2/1(Aero Force) -> Bus Creator1/4  "Damping"
  Dryden Wind Turbulence Model (Discrete (+q +r))/1 -> Sum/2
  Constant/1 -> Bus Creator1/2
  Radians to Degrees/1 -> Abs/1
  Abs/1 -> 2-D Lookup Table1/1

== system FlightSimulation/Flight Dynamics/Mass Update ==
  m_dot : Inport
  Constant : Constant  Value=kins.m_0 + MotorModel.emptyWt + MotorModel.propWt
  Integrator : Integrator
  Sum : Sum  Inputs=|-+
  mass : Outport
  wires:
  m_dot/1 -> Integrator/1
  Integrator/1 -> Sum/1
  Sum/1 -> mass/1
  Constant/1 -> Sum/2

== system FlightSimulation/Flight Dynamics/Motor Model ==
  Time : Inport
  2-D Lookup Table : Lookup_n-D  NumberOfTableDimensions=1  BreakpointsForDimension1=MotorModel.timePts  BreakpointsForDimension2=[1:3]  Table=MotorModel.thrustPts  ExtrapMethod=Clip  ApplyFullPrecisionForLinearInterpolation=on  InternalRulePriority=Speed  RndMeth=Simplest
  Bus Creator : BusCreator  Inputs=3
  Constant : Constant  Value=MotorModel.Isp
  Constant1 : Constant  Value=const.g_e
  Constant2 : Constant  Value=[1;0;0]
  Divide : Product  Inputs=*/
  Product : Product
  Product1 : Product
  MotorBus : Outport
  wires:
  Bus Creator/1 -> MotorBus/1
  Time/1 -> 2-D Lookup Table/1  "Time"
  Product/1 -> Bus Creator/3, Divide/2  "c"
  Constant/1 -> Product/1
  Constant1/1 -> Product/2
  Divide/1 -> Bus Creator/2  "m_dot"
  2-D Lookup Table/1 -> Divide/1, Product1/1  "Thrust"
  Constant2/1 -> Product1/2
  Product1/1 -> Bus Creator/1  "Thrust"

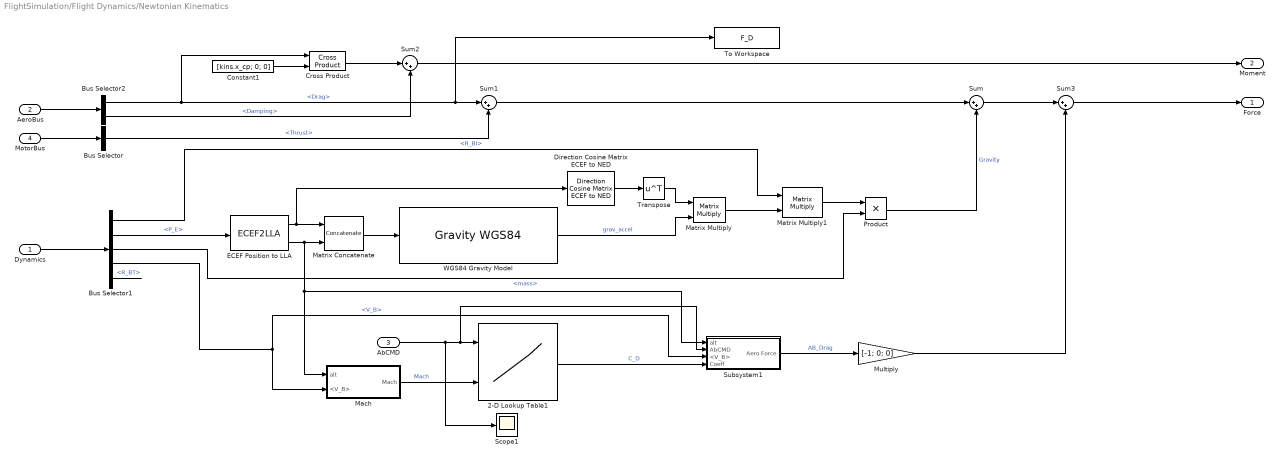
== system FlightSimulation/Flight Dynamics/Newtonian Kinematics ==
  Dynamics : Inport
  AeroBus : Inport  Port=2
  AbCMD : Inport  Port=3
  MotorBus : Inport  Port=4
  2-D Lookup Table1 : Lookup_n-D  BreakpointsForDimension1=AeroModel.AB.PercentActuation  BreakpointsForDimension2=AeroModel.AB.MachNumbers  Table=AeroModel.AB.CdGrid  InternalRulePriority=Speed  RndMeth=Simplest
      settings: InputPortMap=u0,u1
  Bus Selector : BusSelector  OutputSignals=Thrust
  Bus Selector1 : BusSelector  OutputSignals=R_BI,P_E,mass,V_B,R_BT
  Bus Selector2 : BusSelector  OutputSignals=Drag,Damping
  Constant1 : Constant  Value=[kins.x_cp; 0; 0]
  Cross Product : matrix_library/Cross Product
  Direction Cosine Matrix ECEF to NED : aerolibtransform2/Direction Cosine Matrix ECEF to NED
  ECEF Position to LLA : ECEF2LLA
  Mach : Subsystem
  Matrix Concatenate : Concatenate
  Matrix Multiply : Product  Multiplication=Matrix(*)
  Matrix Multiply1 : Product  Multiplication=Matrix(*)
  Multiply : Gain  Gain=[-1; 0; 0]
  Product : Product
  Scope1 : Scope
      settings: ActiveDisplayYMinimum=-1  ActiveDisplayYMaximum=1  DataLoggingVariableName=ScopeData3
  Subsystem1 : Subsystem
  Sum{,1..3} (4 alike) : Sum  Inputs=|++
  To Workspace : ToWorkspace  VariableName=F_D  SaveFormat=Timeseries  SampleTime=-1
  Transpose : Math  Operator=transpose
  "WGS84 Gravity Model  " : GravityWGS84
  Force : Outport
  Moment : Outport  Port=2
  wires:
  MotorBus/1 -> Bus Selector/1
  Dynamics/1 -> Bus Selector1/1
  AeroBus/1 -> Bus Selector2/1
  ECEF Position to LLA/1 -> Direction Cosine Matrix ECEF to NED/1, Matrix Concatenate/1
  ECEF Position to LLA/2 -> Subsystem1/1(alt), Mach/1(alt), Matrix Concatenate/2
  Matrix Concatenate/1 -> "WGS84 Gravity Model  "/1
  "WGS84 Gravity Model  "/1 -> Matrix Multiply/2  "grav_accel"
  Direction Cosine Matrix ECEF to NED/1 -> Transpose/1
  Transpose/1 -> Matrix Multiply/1
  Sum1/1 -> Sum/1
  Bus Selector1/1 -> Matrix Multiply1/1  "<R_BI>"
  Bus Selector1/2 -> ECEF Position to LLA/1  "<P_E>"
  Bus Selector1/3 -> Product/2  "<mass>"
  Matrix Multiply/1 -> Matrix Multiply1/2
  Matrix Multiply1/1 -> Product/1
  Product/1 -> Sum/2  "Gravity"
  Bus Selector/1 -> Sum1/2  "<Thrust>"
  Bus Selector2/1 -> Cross Product/1, To Workspace/1, Sum1/1  "<Drag>"
  Bus Selector2/2 -> Sum2/2  "<Damping>"
  Cross Product/1 -> Sum2/1
  Constant1/1 -> Cross Product/2
  Sum2/1 -> Moment/1
  Bus Selector1/4 -> Subsystem1/3(<V_B>), Mach/2(<V_B>)  "<V_B>"
  2-D Lookup Table1/1 -> Subsystem1/4(Coeff)  "C_D"
  Subsystem1/1(Aero Force) -> Multiply/1  "AB_Drag"
  Sum/1 -> Sum3/1
  Bus Selector1/5 -> ?  "<R_BT>"
  Sum3/1 -> Force/1
  Mach/1(Mach) -> 2-D Lookup Table1/2  "Mach"
  AbCMD/1 -> Scope1/1, Subsystem1/2(AbCMD), 2-D Lookup Table1/1
  Multiply/1 -> Sum3/2

== system FlightSimulation/Flight Computer/ESKF/dt ==
  Clock : Clock
  Subtract : Sum  Inputs=+-
  Unit Delay : UnitDelay  SampleTime=-1  HasFrameUpgradeWarning=on
  dt : Outport
  time : Outport  Port=2
  wires:
  Clock/1 -> time/1, Unit Delay/1, Subtract/1
  Subtract/1 -> dt/1
  Unit Delay/1 -> Subtract/2

== system FlightSimulation/Flight Computer/Sensor Bus/ICM20948 ==
  <a_b> : Inport
  <w_ib_B> : Inport  Port=2
  <R_BT> : Inport  Port=3
  MATLAB Function : MATLAB Function  TreatAsAtomicUnit=on
  MATLAB Function 1 : MATLAB Function  TreatAsAtomicUnit=on
  MATLAB Function 2 : MATLAB Function  TreatAsAtomicUnit=on
  Random Number : RandomNumber
  Random Number1 : RandomNumber
  sf_B_corr : Outport
  sf_B_true : Outport  Port=2
  w_ib_B_corr : Outport  Port=3
  w_ib_B_true : Outport  Port=4
  wires:
  <a_b>/1 -> MATLAB Function/1(a_b)
  <R_BT>/1 -> MATLAB Function/2(R_BT)
  MATLAB Function/1(sf_true) -> sf_B_true/1, MATLAB Function 1/1(sf_true)
  MATLAB Function 1/1(sf_corr) -> sf_B_corr/1
  <w_ib_B>/1 -> MATLAB Function 2/1(gyro_true), w_ib_B_true/1
  MATLAB Function 2/1(gyro_corr) -> w_ib_B_corr/1
  Random Number/1 -> MATLAB Function 1/2(rn)
  Random Number1/1 -> MATLAB Function 2/2(rn)

== system FlightSimulation/Flight Computer/UKF/Initialize Nav ==
  SensorBus : Inport
  Bus Creator : BusCreator  Inputs=7  OutDataTypeStr=Bus: navBus  NonVirtualBus=on
  Constant1 : Constant  Value=navParams.W_m
  Constant2 : Constant  Value=navParams.Q
  Constant3 : Constant  Value=navParams.P
  Constant4 : Constant  Value=navParams.P_min
  Constant5 : Constant  Value=navParams.W_c
  Delay One Step : Delay  DelayLength=1
  Gain : Gain
  Initialize State : Subsystem
  initFlag : Outport
  NavBus : Outport  Port=2  OutDataTypeStr=Bus: navBus
  wires:
  SensorBus/1 -> Initialize State/2(SensorBus)
  Constant4/1 -> Bus Creator/5  "P_min"
  Constant3/1 -> Bus Creator/4  "P"
  Constant2/1 -> Bus Creator/3  "Q"
  Gain/1 -> Bus Creator/2  "x_min"
  Initialize State/1(x_0) -> Gain/1, Bus Creator/1  "x"
  Bus Creator/1 -> NavBus/1
  Initialize State/2(initFlag) -> initFlag/1, Delay One Step/1
  Delay One Step/1 -> Initialize State/1(initFlagLoop)
  Constant1/1 -> Bus Creator/6  "W_m"
  Constant5/1 -> Bus Creator/7  "W_c"

== system FlightSimulation/Flight Computer/UKF/Prediction Step ==
  NavBus : Inport
  SensorBus : Inport  Port=2
  Enable : EnablePort
  Bus Selector : BusSelector  OutputSignals=ICM20948.sf_B_corr,ICM20948.w_ib_B_corr
  MATLAB Function : MATLAB Function  TreatAsAtomicUnit=on
  navOut : Outport
  wires:
  Bus Selector/1 -> MATLAB Function/2(sf_b)  "<sf_B_corr>"
  SensorBus/1 -> Bus Selector/1
  Bus Selector/2 -> MATLAB Function/3(w_ib_b)  "<w_ib_B_corr>"
  NavBus/1 -> MATLAB Function/1(navIn)
  MATLAB Function/1(navOut) -> navOut/1

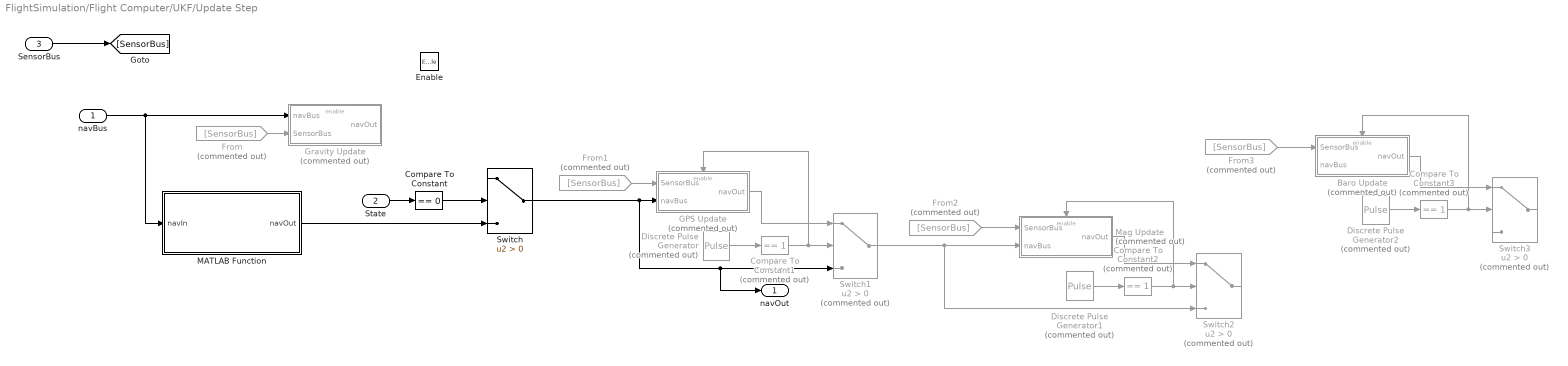
== system FlightSimulation/Flight Computer/UKF/Update Step ==
  navBus : Inport
  State : Inport  Port=2
  SensorBus : Inport  Port=3
  Enable : EnablePort
  Baro Update : Subsystem  Commented=on  TreatAsAtomicUnit=on
  Compare To Constant : simulink/Logic and Bit Operations/Compare To Constant  relop===  const=0  OutDataTypeStr=boolean
  Compare To Constant1 : simulink/Logic and Bit Operations/Compare To Constant  Commented=on  relop===  const=1  OutDataTypeStr=boolean
  Compare To Constant2 : simulink/Logic and Bit Operations/Compare To Constant  Commented=on  relop===  const=1  OutDataTypeStr=boolean
  Compare To Constant3 : simulink/Logic and Bit Operations/Compare To Constant  Commented=on  relop===  const=1  OutDataTypeStr=boolean
  Discrete Pulse Generator : DiscretePulseGenerator  Commented=on  Period=5  SampleTime=time.navDt
  Discrete Pulse Generator1 : DiscretePulseGenerator  Commented=on  Period=5  SampleTime=time.navDt
  Discrete Pulse Generator2 : DiscretePulseGenerator  Commented=on  Amplitude=0  Period=5  SampleTime=time.navDt
  From{,1..3} (4 alike) : From  Commented=on  GotoTag=SensorBus
  GPS Update : Subsystem  Commented=on  TreatAsAtomicUnit=on
  Gravity Update : Subsystem  Commented=on
  MATLAB Function : MATLAB Function  TreatAsAtomicUnit=on
  Mag Update : Subsystem  Commented=on  TreatAsAtomicUnit=on
  Switch : Switch  Criteria=u2 > Threshold  SaturateOnIntegerOverflow=off  InputSameDT=off
  Switch1 : Switch  Commented=on  Criteria=u2 > Threshold  SaturateOnIntegerOverflow=off  InputSameDT=off
  Switch2 : Switch  Commented=on  Criteria=u2 > Threshold  SaturateOnIntegerOverflow=off  InputSameDT=off
  Switch3 : Switch  Commented=on  Criteria=u2 > Threshold  SaturateOnIntegerOverflow=off  InputSameDT=off
  navOut : Outport
  wires:
  navBus/1 -> MATLAB Function/1(navIn), Gravity Update/1(navBus)
  Compare To Constant/1 -> Switch/2
  MATLAB Function/1(navOut) -> Switch/3
  GPS Update/1(navOut) -> Switch1/1
  SensorBus/1 -> [SensorBus]
  From/1 -> Gravity Update/2(SensorBus)
  Discrete Pulse Generator/1 -> Compare To Constant1/1
  Compare To Constant1/1 -> GPS Update/Enable, Switch1/2
  Compare To Constant2/1 -> Mag Update/Enable, Switch2/2
  Discrete Pulse Generator1/1 -> Compare To Constant2/1
  From2/1 -> Mag Update/1(SensorBus)
  Mag Update/1(navOut) -> Switch2/1
  Discrete Pulse Generator2/1 -> Compare To Constant3/1
  Baro Update/1(navOut) -> Switch3/1
  From3/1 -> Baro Update/1(SensorBus)
  Compare To Constant3/1 -> Baro Update/Enable, Switch3/2
  From1/1 -> GPS Update/1(SensorBus)
  Switch1/1 -> Switch2/3, Mag Update/2(navBus)
  Switch/1 -> navOut/1, Switch1/3, GPS Update/2(navBus)
  State/1 -> Compare To Constant/1

== system FlightSimulation/Flight Dynamics/Aero/AoA ==
  Vec_hat : Inport
  Atan : Trigonometry  Operator=atan
  Divide : Product  Inputs=*/
  Selector : Selector  InputPortWidth=3  IndexOptions=Index vector (dialog)  Indices=3  OutputSizes=1
  Selector1 : Selector  InputPortWidth=3  IndexOptions=Index vector (dialog)  Indices=1  OutputSizes=1
  AoA : Outport
  wires:
  Vec_hat/1 -> Selector1/1, Selector/1
  Selector/1 -> Divide/1
  Selector1/1 -> Divide/2
  Divide/1 -> Atan/1  "AoA"
  Atan/1 -> AoA/1

== system FlightSimulation/Flight Dynamics/Aero/Damping ==
  Dynamics : Inport
  Bus Selector : BusSelector  OutputSignals=w_ib_B
  Constant : Constant  Value=-AeroModel.damping.Cd_x*kins.S*kins.x_cp
  Constant1 : Constant  Value=-AeroModel.damping.Cd_y*kins.S*kins.x_cp
  Constant2 : Constant  Value=-AeroModel.damping.Cd_z*kins.S*kins.x_cp
  Product : Product
  Scope : Scope
      settings: ActiveDisplayYMinimum=-0.11753  ActiveDisplayYMaximum=0.06187  DataLoggingVariableName=ScopeData3
  Vector Concatenate : Concatenate  NumInputs=3
  Coeff : Outport
  wires:
  Constant/1 -> Vector Concatenate/1
  Constant1/1 -> Vector Concatenate/2
  Constant2/1 -> Vector Concatenate/3
  Dynamics/1 -> Bus Selector/1
  Bus Selector/1 -> Scope/1, Product/1  "<w_ib_B>"
  Vector Concatenate/1 -> Product/2
  Product/1 -> Coeff/1

== system FlightSimulation/Flight Dynamics/Aero/Mach ==
  <V_B> : Inport
  alt : Inport  Port=2
  Divide : Product  Inputs=*/
  Dot Product1 : DotProduct  OutDataTypeStr=Inherit: Inherit via internal rule
  ISA Atmosphere Model : aerolibatmos2/ISA Atmosphere Model  useExtended=off  action=Warning  custom=off  viscosityOut=off  g=9.80665  gamma=1.4  R=287.0531  L=0.0065  h_trop=11000  h_strat=20000  rho0=1.225  P0=101325  T0=288.15  h0=0  S=110.4  Tref=273.15  muref=1.716e-5
  Sqrt1 : Sqrt
  Terminator : Terminator
  Terminator1 : Terminator
  Terminator2 : Terminator
  Mach : Outport
  wires:
  Dot Product1/1 -> Sqrt1/1
  <V_B>/1 -> Dot Product1/2, Dot Product1/1
  Sqrt1/1 -> Divide/1  "v_B"
  alt/1 -> ISA Atmosphere Model/1
  ISA Atmosphere Model/2 -> Divide/2
  Divide/1 -> Mach/1
  ISA Atmosphere Model/1 -> Terminator/1
  ISA Atmosphere Model/3 -> Terminator1/1
  ISA Atmosphere Model/4 -> Terminator2/1

== system FlightSimulation/Flight Dynamics/Aero/Magnitude ==
  In1 : Inport
  Dot Product : DotProduct  OutDataTypeStr=Inherit: Inherit via internal rule
  Sqrt : Sqrt
  Out1 : Outport
  wires:
  In1/1 -> Dot Product/2, Dot Product/1
  Dot Product/1 -> Sqrt/1
  Sqrt/1 -> Out1/1

== system FlightSimulation/Flight Dynamics/Aero/Subsystem ==
  <V_B> : Inport
  Coeff : Inport  Port=2
  alt : Inport  Port=3
  Constant : Constant  Value=2
  Dot Product1 : DotProduct  OutDataTypeStr=Inherit: Inherit via internal rule
  Gain : Gain  Gain=1/2 * kins.S
  ISA Atmosphere Model : aerolibatmos2/ISA Atmosphere Model  useExtended=off  action=Warning  custom=off  viscosityOut=off  g=9.80665  gamma=1.4  R=287.0531  L=0.0065  h_trop=11000  h_strat=20000  rho0=1.225  P0=101325  T0=288.15  h0=0  S=110.4  Tref=273.15  muref=1.716e-5
  Power : Math  Operator=pow
  Product : Product
  Product1 : Product
  Sqrt1 : Sqrt
  Aero Force : Outport
  wires:
  alt/1 -> ISA Atmosphere Model/1
  ISA Atmosphere Model/4 -> Product1/2
  Dot Product1/1 -> Sqrt1/1
  <V_B>/1 -> Dot Product1/2, Dot Product1/1
  Product/1 -> Aero Force/1
  Coeff/1 -> Product/2
  Sqrt1/1 -> Power/1  "v_B"
  Constant/1 -> Power/2
  Power/1 -> Product1/1
  Product1/1 -> Gain/1
  Gain/1 -> Product/1

== system FlightSimulation/Flight Dynamics/Aero/Subsystem2 ==
  <V_B> : Inport
  Coeff : Inport  Port=2
  alt : Inport  Port=3
  Constant : Constant  Value=2
  Dot Product1 : DotProduct  OutDataTypeStr=Inherit: Inherit via internal rule
  Gain : Gain  Gain=1/2 * kins.S
  ISA Atmosphere Model : aerolibatmos2/ISA Atmosphere Model  useExtended=off  action=Warning  custom=off  viscosityOut=off  g=9.80665  gamma=1.4  R=287.0531  L=0.0065  h_trop=11000  h_strat=20000  rho0=1.225  P0=101325  T0=288.15  h0=0  S=110.4  Tref=273.15  muref=1.716e-5
  Power : Math  Operator=pow
  Product : Product
  Product1 : Product
  Sqrt1 : Sqrt
  Aero Force : Outport
  wires:
  alt/1 -> ISA Atmosphere Model/1
  ISA Atmosphere Model/4 -> Product1/2
  Dot Product1/1 -> Sqrt1/1
  <V_B>/1 -> Dot Product1/2, Dot Product1/1
  Product/1 -> Aero Force/1
  Coeff/1 -> Product/2
  Sqrt1/1 -> Power/1  "v_B"
  Constant/1 -> Power/2
  Power/1 -> Product1/1
  Product1/1 -> Gain/1
  Gain/1 -> Product/1

== system FlightSimulation/Flight Dynamics/Aero/Unit Vector ==
  Vec : Inport
  Divide : Product  Inputs=*/
  Dot Product1 : DotProduct  OutDataTypeStr=Inherit: Inherit via internal rule
  Sqrt1 : Sqrt
  Vec_hat : Outport
  wires:
  Vec/1 -> Divide/1, Dot Product1/2, Dot Product1/1
  Dot Product1/1 -> Sqrt1/1
  Sqrt1/1 -> Divide/2
  Divide/1 -> Vec_hat/1

== system FlightSimulation/Flight Dynamics/Newtonian Kinematics/Mach ==
  alt : Inport
  <V_B> : Inport  Port=2
  Divide : Product  Inputs=*/
  Dot Product1 : DotProduct  OutDataTypeStr=Inherit: Inherit via internal rule
  ISA Atmosphere Model : aerolibatmos2/ISA Atmosphere Model  useExtended=off  action=Warning  custom=off  viscosityOut=off  g=9.80665  gamma=1.4  R=287.0531  L=0.0065  h_trop=11000  h_strat=20000  rho0=1.225  P0=101325  T0=288.15  h0=0  S=110.4  Tref=273.15  muref=1.716e-5
  Scope : Scope
      settings: ActiveDisplayYMinimum=-1  ActiveDisplayYMaximum=1
  Sqrt1 : Sqrt
  Terminator : Terminator
  Terminator1 : Terminator
  Terminator2 : Terminator
  Mach : Outport
  wires:
  Dot Product1/1 -> Sqrt1/1
  <V_B>/1 -> Dot Product1/2, Dot Product1/1
  Sqrt1/1 -> Divide/1  "v_B"
  alt/1 -> Scope/1, ISA Atmosphere Model/1
  ISA Atmosphere Model/2 -> Divide/2
  Divide/1 -> Mach/1
  ISA Atmosphere Model/1 -> Terminator/1
  ISA Atmosphere Model/3 -> Terminator1/1
  ISA Atmosphere Model/4 -> Terminator2/1

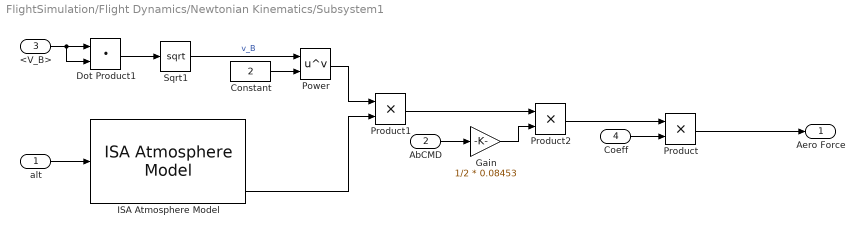
== system FlightSimulation/Flight Dynamics/Newtonian Kinematics/Subsystem1 ==
  alt : Inport
  AbCMD : Inport  Port=2
  <V_B> : Inport  Port=3
  Coeff : Inport  Port=4
  Constant : Constant  Value=2
  Dot Product1 : DotProduct  OutDataTypeStr=Inherit: Inherit via internal rule
  Gain : Gain  Gain=1/2 * 0.08453
  ISA Atmosphere Model : aerolibatmos2/ISA Atmosphere Model  useExtended=off  action=Warning  custom=off  viscosityOut=off  g=9.80665  gamma=1.4  R=287.0531  L=0.0065  h_trop=11000  h_strat=20000  rho0=1.225  P0=101325  T0=288.15  h0=0  S=110.4  Tref=273.15  muref=1.716e-5
  Power : Math  Operator=pow
  Product : Product
  Product1 : Product
  Product2 : Product
  Sqrt1 : Sqrt
  Aero Force : Outport
  wires:
  alt/1 -> ISA Atmosphere Model/1
  ISA Atmosphere Model/4 -> Product1/2
  Dot Product1/1 -> Sqrt1/1
  <V_B>/1 -> Dot Product1/2, Dot Product1/1
  Product/1 -> Aero Force/1
  Coeff/1 -> Product/2
  Sqrt1/1 -> Power/1  "v_B"
  Constant/1 -> Power/2
  Power/1 -> Product1/1
  AbCMD/1 -> Gain/1
  Product1/1 -> Product2/1
  Gain/1 -> Product2/2
  Product2/1 -> Product/1

== system FlightSimulation/Flight Computer/UKF/Initialize Nav/Initialize State ==
  initFlagLoop : Inport
  SensorBus : Inport  Port=2
  Bus Selector2 : BusSelector  OutputSignals=ICM20948.sf_B_corr,MMC5983.B_corr
  MATLAB Function1 : MATLAB Function  TreatAsAtomicUnit=on
  MATLAB Function2 : MATLAB Function  Commented=on  TreatAsAtomicUnit=on
  MATLAB Function3 : MATLAB Function  Commented=on  TreatAsAtomicUnit=on
  MATLAB Function4 : MATLAB Function  TreatAsAtomicUnit=on
  x_0 : Outport
  initFlag : Outport  Port=2
  wires:
  SensorBus/1 -> Bus Selector2/1
  MATLAB Function2/1(q_0) -> MATLAB Function3/2(q_0)  "q_0"
  Bus Selector2/1 -> MATLAB Function1/1(a_b)  "<sf_B_corr>"
  Bus Selector2/2 -> MATLAB Function1/2(m_b)  "<B_corr>"
  MATLAB Function1/1(eul_0) -> MATLAB Function4/2(eul_0)  "eul_0"
  initFlagLoop/1 -> MATLAB Function4/1(initFlagLoop)
  MATLAB Function4/1(x_0) -> x_0/1
  MATLAB Function4/2(initFlag) -> initFlag/1

== system FlightSimulation/Flight Computer/UKF/Update Step/Baro Update ==
  SensorBus : Inport
  navBus : Inport  Port=2
  Enable : EnablePort
  Bus Selector : BusSelector  OutputSignals=LPS22.P_corr
  MATLAB Function : MATLAB Function  TreatAsAtomicUnit=on
  navOut : Outport
  wires:
  MATLAB Function/1(navOut) -> navOut/1
  navBus/1 -> MATLAB Function/1(navIn)
  SensorBus/1 -> Bus Selector/1
  Bus Selector/1 -> MATLAB Function/2(u_baro)  "<P_corr>"
